simulink model "motor_tf_verification"  (R2018a)
settings: Solver=ode23tb  StartTime=0.0  StopTime=3  FixedStep=1274.587e-6  RelTol=1e-3
values from neighbouring files (symbols this model uses):
  b = 0.01    [Values.m]
undefined symbols (not defined in the file or in its folder): data, Ip
libraries: dspsrcs4 x4
settings Model: Creator=gokarna  LastModifiedBy=devko

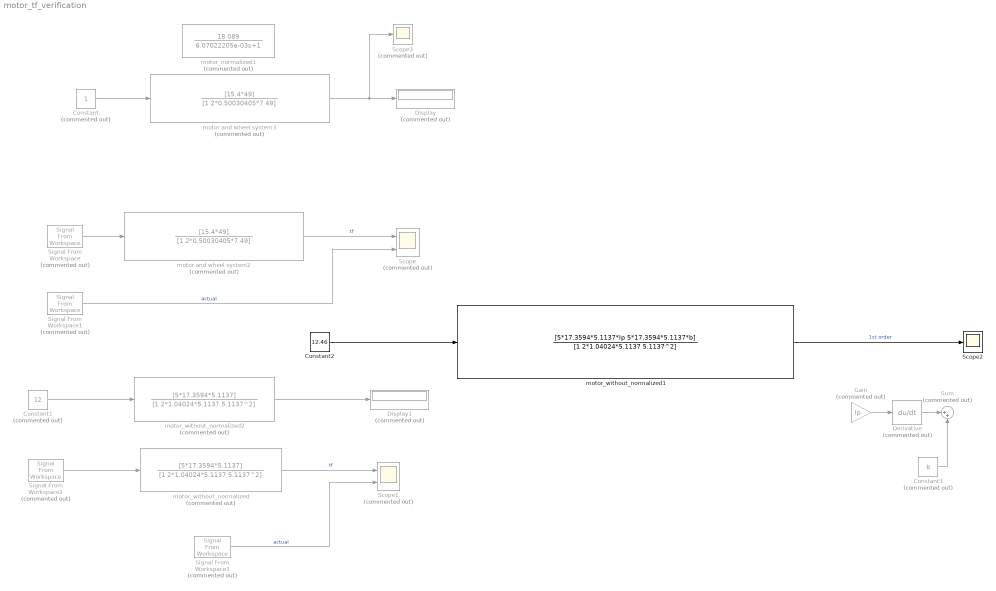
== system motor_tf_verification ==
  Constant : Constant  Commented=on
  Constant1 : Constant  Commented=on  Value=12
  Constant2 : Constant  Value=12.46
  Constant3 : Constant  Commented=on  Value=b
  Derivative : Derivative  Commented=on
  Display : Display  Commented=on
  Display1 : Display  Commented=on
  Gain : Gain  Commented=on  Gain=Ip
  Scope : Scope  Commented=on  NumInputPorts=2
  Scope1 : Scope  Commented=on  NumInputPorts=2
  Scope2 : Scope
  Scope3 : Scope  Commented=on
  Signal From Workspace : dspsrcs4/Signal From Workspace  Commented=on  X=voltage  Ts=1  nsamps=1  OutputAfterFinalValue=Setting to zero  ignoreOrWarnInputAndFrameLengths=off  OutputFrames=off
  Signal From Workspace1 : dspsrcs4/Signal From Workspace  Commented=on  X=rpm  Ts=1  nsamps=1  OutputAfterFinalValue=Setting to zero  ignoreOrWarnInputAndFrameLengths=off  OutputFrames=off
  Signal From Workspace2 : dspsrcs4/Signal From Workspace  Commented=on  X=data(2,:)  Ts=1  nsamps=1  OutputAfterFinalValue=Setting to zero  ignoreOrWarnInputAndFrameLengths=off  OutputFrames=off
  Signal From Workspace3 : dspsrcs4/Signal From Workspace  Commented=on  X=data(3,:)  Ts=1  nsamps=1  OutputAfterFinalValue=Setting to zero  ignoreOrWarnInputAndFrameLengths=off  OutputFrames=off
  Sum : Sum  Commented=on  Inputs=|++
  motor and wheel system2 : TransferFcn  Commented=on  Numerator=[15.4*49]  Denominator=[1 2*0.50030405*7 49]
  motor and wheel system3 : TransferFcn  Commented=on  Numerator=[15.4*49]  Denominator=[1 2*0.50030405*7 49]
  motor_normalized1 : TransferFcn  Commented=on  Numerator=[18.089]  Denominator=[6.07022205e-03 1]
  motor_without_normalized : TransferFcn  Commented=on  Numerator=[5*17.3594*5.1137]  Denominator=[1 2*1.04024*5.1137 5.1137^2]
  motor_without_normalized1 : TransferFcn  Numerator=[5*17.3594*5.1137*Ip 5*17.3594*5.1137*b]  Denominator=[1 2*1.04024*5.1137 5.1137^2]
  motor_without_normalized2 : TransferFcn  Commented=on  Numerator=[5*17.3594*5.1137]  Denominator=[1 2*1.04024*5.1137 5.1137^2]
  wires:
  Signal From Workspace/1 -> motor and wheel system2/1
  motor and wheel system2/1 -> Scope/1  "tf"
  Signal From Workspace1/1 -> Scope/2  "actual"
  Signal From Workspace2/1 -> motor_without_normalized/1
  motor_without_normalized/1 -> Scope1/1  "tf"
  Signal From Workspace3/1 -> Scope1/2  "actual"
  motor and wheel system3/1 -> Scope3/1, Display/1
  Constant/1 -> motor and wheel system3/1
  Constant1/1 -> motor_without_normalized2/1
  motor_without_normalized2/1 -> Display1/1
  motor_without_normalized1/1 -> Scope2/1  "1st order"
  Gain/1 -> Derivative/1
  Derivative/1 -> Sum/1
  Constant3/1 -> Sum/2
  Constant2/1 -> motor_without_normalized1/1
